simulink model "exercicio1"  (R2019a)
settings: Solver=FixedStepAuto  StartTime=0.0  StopTime=50  FixedStep=1e-3  RelTol=1e-3
undefined symbols (not defined in the file): a1, a2, C, controle, r, R
libraries: simulink x2
settings Model: Creator=guilh  LastModifiedBy=guilh
settings DataIOCC: SaveOutput=off  SignalLogging=off  DSMLogging=off  ReturnWorkspaceOutputs=off  TimeSaveName=t

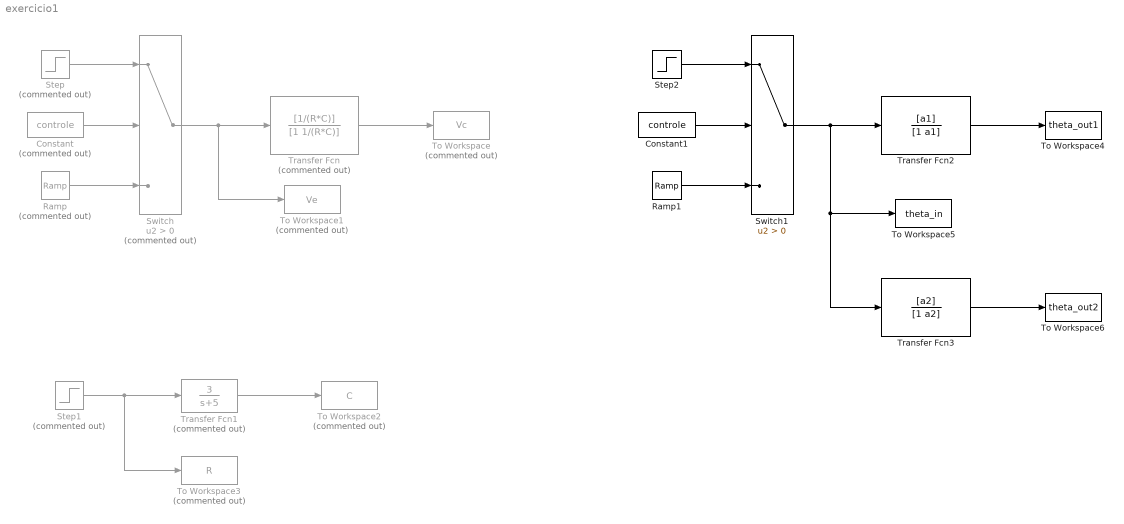
== system exercicio1 ==
  Constant : Constant  Commented=on  Value=controle
  Constant1 : Constant  Value=controle
  Ramp : simulink/Sources/Ramp  Commented=on  slope=3  start=0  InitialOutput=0
  Ramp1 : simulink/Sources/Ramp  slope=r  start=0  InitialOutput=0
  Step : Step  Commented=on  Time=0  After=5  SampleTime=0
  Step1 : Step  Commented=on  Time=0  After=2  SampleTime=0
  Step2 : Step  Time=0  After=r  SampleTime=0
  Switch : Switch  Commented=on  Criteria=u2 > Threshold
  Switch1 : Switch  Criteria=u2 > Threshold
  To Workspace : ToWorkspace  Commented=on  VariableName=Vc  SampleTime=-1
  To Workspace1 : ToWorkspace  Commented=on  VariableName=Ve  SampleTime=-1
  To Workspace2 : ToWorkspace  Commented=on  VariableName=C  SampleTime=-1
  To Workspace3 : ToWorkspace  Commented=on  VariableName=R  SampleTime=-1
  To Workspace4 : ToWorkspace  VariableName=theta_out1  SampleTime=-1
  To Workspace5 : ToWorkspace  VariableName=theta_in  SampleTime=-1
  To Workspace6 : ToWorkspace  VariableName=theta_out2  SampleTime=-1
  Transfer Fcn : TransferFcn  Commented=on  Numerator=[1/(R*C)]  Denominator=[1 1/(R*C)]
  Transfer Fcn1 : TransferFcn  Commented=on  Numerator=[3]  Denominator=[1 5]
  Transfer Fcn2 : TransferFcn  Numerator=[a1]  Denominator=[1 a1]
  Transfer Fcn3 : TransferFcn  Numerator=[a2]  Denominator=[1 a2]
  wires:
  Ramp/1 -> Switch/3
  Step/1 -> Switch/1
  Constant/1 -> Switch/2
  Switch/1 -> To Workspace1/1, Transfer Fcn/1
  Transfer Fcn/1 -> To Workspace/1
  Transfer Fcn1/1 -> To Workspace2/1
  Step1/1 -> To Workspace3/1, Transfer Fcn1/1
  Ramp1/1 -> Switch1/3
  Switch1/1 -> Transfer Fcn3/1, To Workspace5/1, Transfer Fcn2/1
  Step2/1 -> Switch1/1
  Constant1/1 -> Switch1/2
  Transfer Fcn2/1 -> To Workspace4/1
  Transfer Fcn3/1 -> To Workspace6/1
